simulink model "hw3"  (R2013a)
settings: Solver=ode45  StartTime=0.0  StopTime=20  RelTol=1e-3
settings Model: Creator=bazkoale  LastModifiedBy=bazkoale

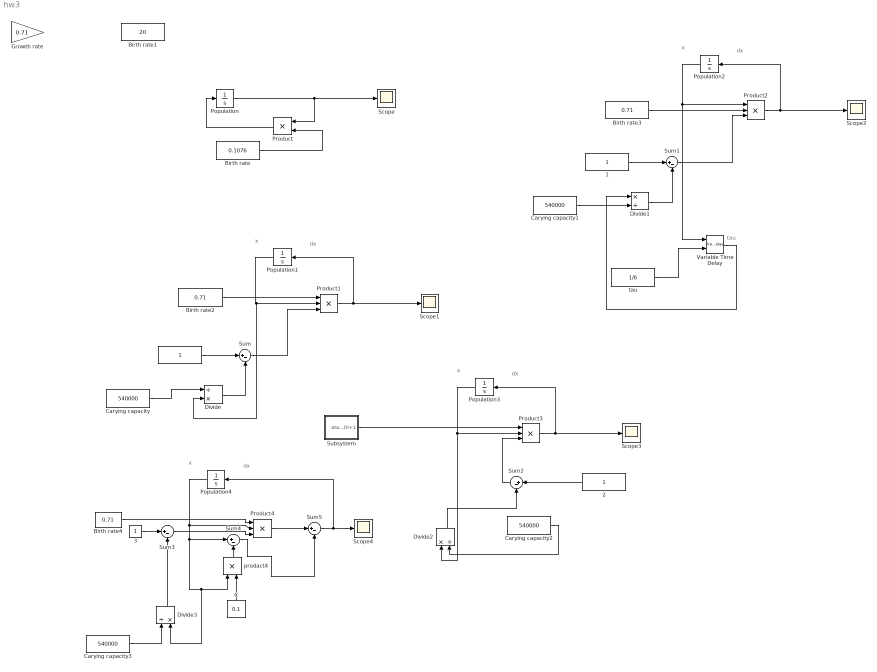
== system hw3 ==
  note: tau
  note: x
  note: dx
  note: x
  note: dx
  note: x
  note: dx
  note: x
  note: dx
   {,1..3} (4 alike) : Constant
  " tau" : Constant  Value=1/6
  Birth rate : Constant  Value=0.1076
  Birth rate1 : Constant  Value=20
  Birth rate2 : Constant  Value=0.71
  Birth rate3 : Constant  Value=0.71
  Birth rate4 : Constant  Value=0.71
  C : Constant  Value=0.1
  Carying capacity{,1..3} (4 alike) : Constant  Value=540000
  Divide : Product  Inputs=/*
  Divide1 : Product  Inputs=*/
  Divide2 : Product  Inputs=*/
  Divide3 : Product  Inputs=/*
  Growth rate : Gain  Gain=0.71
  Population : Integrator  InitialCondition=14.4775
  Population{1..4} (4 alike) : Integrator  InitialCondition=540000/4
  Product : Product
  Product{1..4} (4 alike) : Product  Inputs=3
  Scope{,1..4} (5 alike) : Scope
      Scope2 settings: SaveName=ScopeData2
      Scope3 settings: SaveName=ScopeData3
      Scope4 settings: SaveName=ScopeData4
  Subsystem : Subsystem
  Sum{,1..5} (6 alike) : Sum  Inputs=|+-
  Variable Time Delay : VariableTransportDelay  MaximumDelay=10
  "prodact4 " : Product  Inputs=**
  wires:
  Population/1 -> Scope/1, Product/1
  Birth rate/1 -> Product/2
  Product/1 -> Population/1
  Population1/1 -> Divide/2, Product1/2
  " "/1 -> Sum/1
  Divide/1 -> Sum/2
  Product1/1 -> Scope1/1, Population1/1
  Population2/1 -> Variable Time Delay/1, Product2/1
  Birth rate3/1 -> Product2/2
  " 1"/1 -> Sum1/1
  Carying capacity1/1 -> Divide1/2
  Divide1/1 -> Sum1/2
  Sum1/1 -> Product2/3
  Product2/1 -> Scope2/1, Population2/1
  " tau"/1 -> Variable Time Delay/2
  Birth rate2/1 -> Product1/1
  Variable Time Delay/1 -> Divide1/1
  Sum/1 -> Product1/3
  Population3/1 -> Product3/2, Divide2/1
  Carying capacity2/1 -> Divide2/2
  Divide2/1 -> Sum2/2
  Product3/1 -> Population3/1, Scope3/1
  Sum2/1 -> Product3/3
  Subsystem/1("atan(1/t)+1 ") -> Product3/1
  " 2"/1 -> Sum2/1
  Population4/1 -> Divide3/2, "prodact4 "/1, Sum4/1, Product4/2
  " 3"/1 -> Sum3/1
  Divide3/1 -> Sum3/2
  Birth rate4/1 -> Product4/1
  Sum3/1 -> Product4/3
  "prodact4 "/1 -> Sum4/2
  C/1 -> "prodact4 "/2
  Carying capacity3/1 -> Divide3/1
  Sum4/1 -> Sum5/2
  Sum5/1 -> Population4/1, Scope4/1
  Product4/1 -> Sum5/1
  Carying capacity/1 -> Divide/1

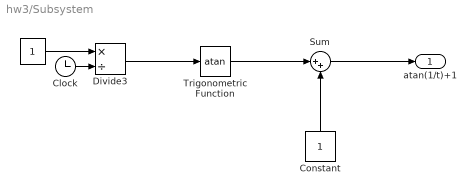
== system hw3/Subsystem ==
  " " : Constant
  Clock : Clock
  Constant : Constant
  Divide3 : Product  Inputs=*/
  Sum : Sum  Inputs=|++
  Trigonometric Function : Trigonometry  Operator=atan
  "atan(1/t)+1 " : Outport
  wires:
  " "/1 -> Divide3/1
  Clock/1 -> Divide3/2
  Divide3/1 -> Trigonometric Function/1
  Trigonometric Function/1 -> Sum/1
  Constant/1 -> Sum/2
  Sum/1 -> "atan(1/t)+1 "/1
